simulink model "tanquesimples"  (R2016a)
settings: Solver=VariableStepAuto  StartTime=0.0  StopTime=20  RelTol=1e-3
libraries: simulink x1
settings Model: Creator=Ítalo Renan  LastModifiedBy=Ítalo Renan

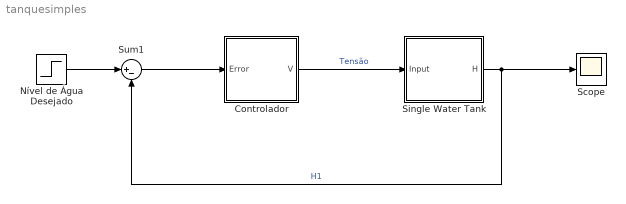
== system tanquesimples ==
  Controlador : Subsystem
  Nível de Água Desejado : Step  Before=14  After=15  SampleTime=0.01
  Scope : Scope
  Single Water Tank : Subsystem
  Sum1 : Sum  Inputs=|+-  SaturateOnIntegerOverflow=on
  wires:
  Nível de Água Desejado/1 -> Sum1/1
  Single Water Tank/1(H) -> Sum1/2, Scope/1  "H1"
  Sum1/1 -> Controlador/1(Error)
  Controlador/1(V) -> Single Water Tank/1(Input)  "Tensão"

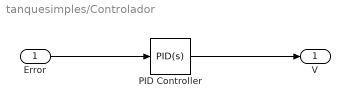
== system tanquesimples/Controlador ==
  Error : Inport
  PID Controller : simulink/Continuous/PID Controller  Tag=PID1  Controller=PID  TimeDomain=Continuous-time  SampleTime=-1  IntegratorMethod=Forward Euler  FilterMethod=Forward Euler  Form=Parallel  UseFilter=off  ControllerParametersSource=internal  P=20  I=0  D=0  N=1  InitialConditionSource=internal  InitialConditionForIntegrator=1.2649  InitialConditionForFilter=0  ExternalReset=none  ZeroCross=off  LimitOutput=off  UpperSaturationLimit=inf  LowerSaturationLimit=-inf  LinearizeAsGain=off  AntiWindupMode=none  Kb=1  TrackingMode=off  Kt=1  PParamMin=[ ]  PParamMax=[ ]  IParamMin=[ ]  IParamMax=[ ]  DParamMin=[ ]  DParamMax=[ ]  NParamMin=[ ]  NParamMax=[ ]  KbParamMin=[ ]  KbParamMax=[ ]  KtParamMin=[ ]  KtParamMax=[ ]  POutMin=[ ]  POutMax=[ ]  IOutMin=[ ]  IOutMax=[ ]  DOutMin=[ ]  DOutMax=[ ]  NOutMin=[ ]  NOutMax=[ ]  KbOutMin=[ ]  KbOutMax=[ ]  KtOutMin=[ ]  KtOutMax=[ ]  IntegratorOutMin=[ ]  IntegratorOutMax=[ ]  FilterOutMin=[ ]  FilterOutMax=[ ]  SumOutMin=[ ]  SumOutMax=[ ]  SumI1OutMin=[ ]  SumI1OutMax=[ ]  SumI2OutMin=[ ]  SumI2OutMax=[ ]  SumI3OutMin=[ ]  SumI3OutMax=[ ]  SumDOutMin=[ ]  SumDOutMax=[ ]  SaturationOutMin=[ ]  SaturationOutMax=[ ]  IntegratorContinuousStateAttributes=''  IntegratorStateMustResolveToSignalObject=off  IntegratorRTWStateStorageClass=Auto  FilterContinuousStateAttributes=''  FilterStateMustResolveToSignalObject=off  FilterRTWStateStorageClass=Auto  DifferentiatorICPrevScaledInput=0  DifferentiatorOutMin=[]  DifferentiatorOutMax=[]
  V : Outport
  wires:
  Error/1 -> PID Controller/1
  PID Controller/1 -> V/1

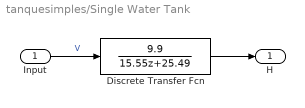
== system tanquesimples/Single Water Tank ==
  Input : Inport
  Discrete Transfer Fcn : DiscreteTransferFcn  Numerator=[9.9]  Denominator=[15.55 25.49]
  H : Outport
  wires:
  Discrete Transfer Fcn/1 -> H/1
  Input/1 -> Discrete Transfer Fcn/1  "V"
